simulink subsystem "FlipHDL"  (R2024b)
settings: Solver=VariableStepAuto  StartTime=0.0  StopTime=10.0  RelTol=1e-3
model mask{flipAlong=Rows}
  mask prompts: flipAlong "Flip Along"
settings Model: Creator=stefano  LastModifiedBy=stefano

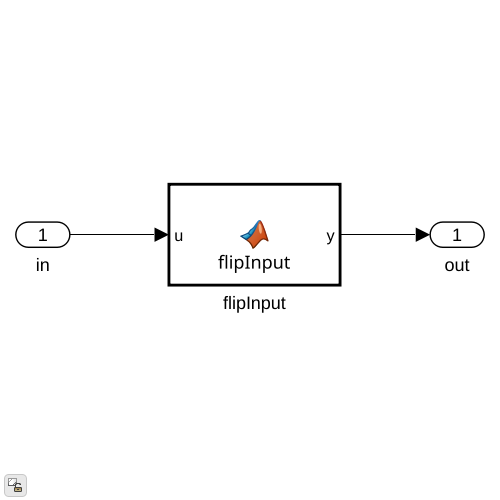
[thumbnail: Simulink's stored preview of the top-level diagram]
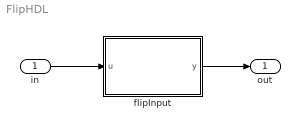
== system FlipHDL ==
  in : Inport
  flipInput : MATLAB Function  TreatAsAtomicUnit=on
  out : Outport
  wires:
  in/1 -> flipInput/1(u)
  flipInput/1(y) -> out/1

== matlab function FlipHDL/flipInput ==
  data: u input; y output; flipAlong parameter
function y = flipInput(u, flipAlong)
    
    y = zeros(size(u), "like", u);

    switch flipAlong
        case 1
            for iElement = 1:size(u, 2)
                y(:, iElement) = u(:, size(u, 2) - iElement + 1);
            end
        case 2
            for iElement = 1:size(u, 1)
                y(iElement, :) = u(size(u, 1) - iElement + 1, :);
            end
    end
end
